simulink model "ctrl_stab"  (R2014b)
settings: Solver=ode45  StartTime=0.0  StopTime=7  FixedStep=0.01  MaxStep=1e-3  MinStep=1e-5  RelTol=1e-3
PreLoadFcn:
  | load('imu_yaw');
libraries: simulink x2, slident x1
settings Model: Creator=Ugo Pattacini  LastModifiedBy=Ugo Pattacini
settings DebuggingCC: UnderspecifiedInitializationDetection=Classic  MergeDetectMultiDrivingBlocksExec=none

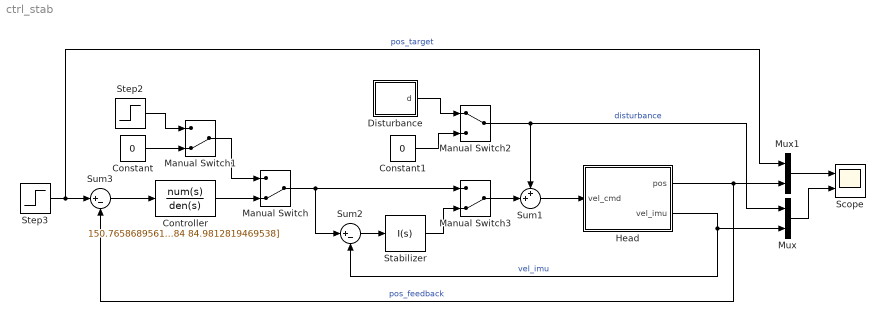
== system ctrl_stab ==
  Constant : Constant  Value=0
  Constant1 : Constant  Value=0
  Controller : TransferFcn  Numerator=150.765868956161  Denominator=[1 15.9669610709384 84.9812819469538]
  Disturbance : Subsystem  mask{t0=1.5, T=3, A=-1}
      mask prompts: t0 "Start Time"; T "Duration"; A "Amplitude"
  Head : Subsystem
  Manual Switch : ManualSwitch  CurrentSetting=0
  Manual Switch1 : ManualSwitch  CurrentSetting=0
  Manual Switch2 : ManualSwitch
  Manual Switch3 : ManualSwitch  CurrentSetting=0
  Mux : Mux  Inputs=2
  Mux1 : Mux  Inputs=2
  Scope : Scope  NumInputPorts=2
      settings: ShowLegends=on  YMin=-5~-5  YMax=5~5
  Stabilizer : simulink/Continuous/PID Controller  Controller=I  TimeDomain=Continuous-time  SampleTime=-1  IntegratorMethod=Trapezoidal  FilterMethod=Trapezoidal  Form=Parallel  P=0  I=11.688043955313  D=0  N=100  InitialConditionSource=internal  InitialConditionForIntegrator=0  InitialConditionForFilter=0  ExternalReset=none  LimitOutput=off  UpperSaturationLimit=inf  LowerSaturationLimit=-inf  LinearizeAsGain=off  AntiWindupMode=none  Kb=1  TrackingMode=off  Kt=1  PParamMin=[]  PParamMax=[]  IParamMin=[]  IParamMax=[]  DParamMin=[]  DParamMax=[]  NParamMin=[]  NParamMax=[]  KbParamMin=[]  KbParamMax=[]  KtParamMin=[]  KtParamMax=[]  POutMin=[]  POutMax=[]  IOutMin=[]  IOutMax=[]  DOutMin=[]  DOutMax=[]  NOutMin=[]  NOutMax=[]  KbOutMin=[]  KbOutMax=[]  KtOutMin=[]  KtOutMax=[]  IntegratorOutMin=[]  IntegratorOutMax=[]  FilterOutMin=[]  FilterOutMax=[]  SumOutMin=[]  SumOutMax=[]  SumI1OutMin=[]  SumI1OutMax=[]  SumI2OutMin=[]  SumI2OutMax=[]  SumI3OutMin=[]  SumI3OutMax=[]  SumDOutMin=[]  SumDOutMax=[]  SaturationOutMin=[]  SaturationOutMax=[]  IntegratorContinuousStateAttributes=''  IntegratorStateMustResolveToSignalObject=off  IntegratorRTWStateStorageClass=Auto  FilterContinuousStateAttributes=''  FilterStateMustResolveToSignalObject=off  FilterRTWStateStorageClass=Auto  DifferentiatorICPrevScaledInput=0  DifferentiatorOutMin=[]  DifferentiatorOutMax=[]  UseFilter=on
  Step2 : Step  Time=2  SampleTime=0
  Step3 : Step  SampleTime=0
  Sum1 : Sum  Inputs=++|
  Sum2 : Sum  Inputs=|+-
  Sum3 : Sum  Inputs=|+-
  wires:
  Sum1/1 -> Head/1(vel_cmd)
  Sum2/1 -> Stabilizer/1
  Head/2(vel_imu) -> Mux/2, Sum2/2  "vel_imu"
  Manual Switch/1 -> Manual Switch3/1, Sum2/1
  Controller/1 -> Manual Switch/2
  Sum3/1 -> Controller/1
  Head/1(pos) -> Mux1/2, Sum3/2  "pos_feedback"
  Manual Switch1/1 -> Manual Switch/1
  Constant/1 -> Manual Switch1/2
  Step2/1 -> Manual Switch1/1
  Mux/1 -> Scope/2
  Mux1/1 -> Scope/1
  Step3/1 -> Mux1/1, Sum3/1  "pos_target"
  Constant1/1 -> Manual Switch2/2
  Disturbance/1(d) -> Manual Switch2/1
  Manual Switch2/1 -> Mux/1, Sum1/1  "disturbance"
  Manual Switch3/1 -> Sum1/2
  Stabilizer/1 -> Manual Switch3/2

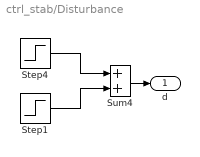
== system ctrl_stab/Disturbance ==
  Step1 : Step  Time=t0+T  After=-A  SampleTime=0
  Step4 : Step  Time=t0  After=A  SampleTime=0
  Sum4 : Sum
  d : Outport
  wires:
  Sum4/1 -> d/1
  Step4/1 -> Sum4/1
  Step1/1 -> Sum4/2

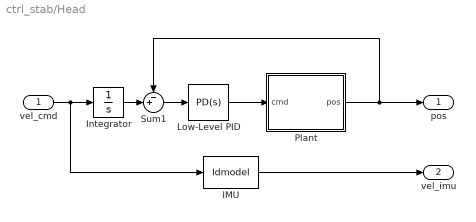
== system ctrl_stab/Head ==
  vel_cmd : Inport
  "IMU " : slident/Models/Idmodel  sys=imu_yaw  IC=0  noi=off  seed=[]
  Integrator : Integrator
  Low-Level PID : simulink/Continuous/PID Controller  Controller=PD  TimeDomain=Continuous-time  SampleTime=-1  IntegratorMethod=Trapezoidal  FilterMethod=Trapezoidal  Form=Parallel  P=122.195125158059  I=1  D=53.9650314282148  N=94.0864796738016  InitialConditionSource=internal  InitialConditionForIntegrator=0  InitialConditionForFilter=0  ExternalReset=none  LimitOutput=off  UpperSaturationLimit=inf  LowerSaturationLimit=-inf  LinearizeAsGain=off  AntiWindupMode=none  Kb=1  TrackingMode=off  Kt=1  PParamMin=[]  PParamMax=[]  IParamMin=[]  IParamMax=[]  DParamMin=[]  DParamMax=[]  NParamMin=[]  NParamMax=[]  KbParamMin=[]  KbParamMax=[]  KtParamMin=[]  KtParamMax=[]  POutMin=[]  POutMax=[]  IOutMin=[]  IOutMax=[]  DOutMin=[]  DOutMax=[]  NOutMin=[]  NOutMax=[]  KbOutMin=[]  KbOutMax=[]  KtOutMin=[]  KtOutMax=[]  IntegratorOutMin=[]  IntegratorOutMax=[]  FilterOutMin=[]  FilterOutMax=[]  SumOutMin=[]  SumOutMax=[]  SumI1OutMin=[]  SumI1OutMax=[]  SumI2OutMin=[]  SumI2OutMax=[]  SumI3OutMin=[]  SumI3OutMax=[]  SumDOutMin=[]  SumDOutMax=[]  SaturationOutMin=[]  SaturationOutMax=[]  IntegratorContinuousStateAttributes=''  IntegratorStateMustResolveToSignalObject=off  IntegratorRTWStateStorageClass=Auto  FilterContinuousStateAttributes=''  FilterStateMustResolveToSignalObject=off  FilterRTWStateStorageClass=Auto  DifferentiatorICPrevScaledInput=0  DifferentiatorOutMin=[]  DifferentiatorOutMax=[]  UseFilter=on
  Plant : Subsystem
  Sum1 : Sum  Inputs=-+|
  pos : Outport
  vel_imu : Outport  Port=2
  wires:
  Integrator/1 -> Sum1/2
  vel_cmd/1 -> "IMU "/1, Integrator/1
  Low-Level PID/1 -> Plant/1(cmd)
  "IMU "/1 -> vel_imu/1
  Sum1/1 -> Low-Level PID/1
  Plant/1(pos) -> Sum1/1, pos/1

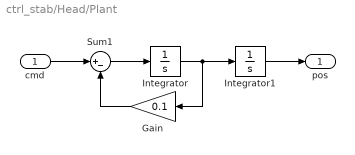
== system ctrl_stab/Head/Plant ==
  cmd : Inport
  Gain : Gain  Gain=0.1
  Integrator : Integrator
  Integrator1 : Integrator
  Sum1 : Sum  Inputs=|+-
  pos : Outport
  wires:
  Integrator/1 -> Gain/1, Integrator1/1
  Sum1/1 -> Integrator/1
  Integrator1/1 -> pos/1
  cmd/1 -> Sum1/1
  Gain/1 -> Sum1/2
